simulink subsystem "PackSOC"  (R2021a)
settings: Solver=VariableStepAuto  StartTime=0.0  StopTime=10.0  RelTol=1e-3
undefined symbols (not defined in the file): CDCEstimation, EKFEstimation
settings Model: Creator=mirko  LastModifiedBy=mirko

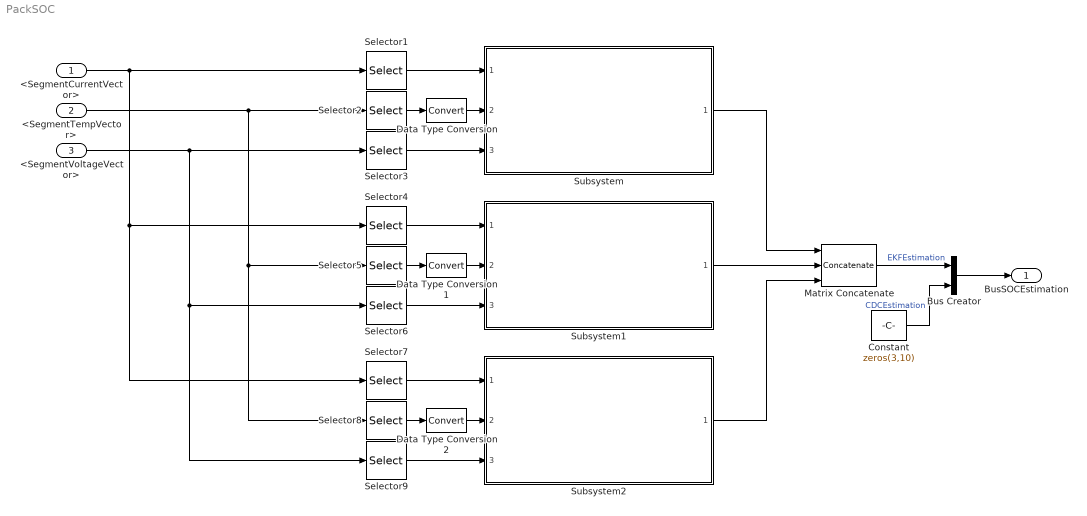
== system PackSOC ==
  <SegmentCurrentVector> : Inport
  <SegmentTempVector> : Inport  Port=2
  <SegmentVoltageVector> : Inport  Port=3
  Bus Creator : BusCreator  Inputs=EKFEstimation,CDCEstimation  OutDataTypeStr=Bus: BusSOCEstimation
  Constant : Constant  Value=zeros(3,10)
  Data Type Conversion : DataTypeConversion
  Data Type Conversion1 : DataTypeConversion
  Data Type Conversion2 : DataTypeConversion
  Matrix Concatenate : Concatenate  NumInputs=3  Mode=Multidimensional array
  Selector1 : Selector  NumberOfDimensions=2  InputPortWidth=3  IndexOptions=Index vector (dialog),Index vector (dialog)  Indices=1,[1 2 3 4 5 6 7 8 9 10]  OutputSizes=1,1
  Selector2 : Selector  NumberOfDimensions=2  InputPortWidth=3  IndexOptions=Index vector (dialog),Index vector (dialog)  Indices=1,[1 2 3 4 5 6 7 8 9 10]  OutputSizes=1,1
  Selector3 : Selector  NumberOfDimensions=2  InputPortWidth=3  IndexOptions=Index vector (dialog),Index vector (dialog)  Indices=1,[1 2 3 4 5 6 7 8 9 10]  OutputSizes=1,1
  Selector4 : Selector  NumberOfDimensions=2  InputPortWidth=3  IndexOptions=Index vector (dialog),Index vector (dialog)  Indices=2,[1 2 3 4 5 6 7 8 9 10]  OutputSizes=1,1
  Selector5 : Selector  NumberOfDimensions=2  InputPortWidth=3  IndexOptions=Index vector (dialog),Index vector (dialog)  Indices=2,[1 2 3 4 5 6 7 8 9 10]  OutputSizes=1,1
  Selector6 : Selector  NumberOfDimensions=2  InputPortWidth=3  IndexOptions=Index vector (dialog),Index vector (dialog)  Indices=2,[1 2 3 4 5 6 7 8 9 10]  OutputSizes=1,1
  Selector7 : Selector  NumberOfDimensions=2  InputPortWidth=3  IndexOptions=Index vector (dialog),Index vector (dialog)  Indices=3,[1 2 3 4 5 6 7 8 9 10]  OutputSizes=1,1
  Selector8 : Selector  NumberOfDimensions=2  InputPortWidth=3  IndexOptions=Index vector (dialog),Index vector (dialog)  Indices=3,[1 2 3 4 5 6 7 8 9 10]  OutputSizes=1,1
  Selector9 : Selector  NumberOfDimensions=2  InputPortWidth=3  IndexOptions=Index vector (dialog),Index vector (dialog)  Indices=3,[1 2 3 4 5 6 7 8 9 10]  OutputSizes=1,1
  Subsystem : Subsystem  ReferencedSubsystem=SegmentSOC
  Subsystem1 : Subsystem  ReferencedSubsystem=SegmentSOC
  Subsystem2 : Subsystem  ReferencedSubsystem=SegmentSOC
  BusSOCEstimation : Outport
  wires:
  <SegmentCurrentVector>/1 -> Selector1/1, Selector7/1, Selector4/1
  <SegmentTempVector>/1 -> Selector2/1, Selector5/1, Selector8/1
  <SegmentVoltageVector>/1 -> Selector3/1, Selector6/1, Selector9/1
  Selector1/1 -> Subsystem/1
  Selector3/1 -> Subsystem/3
  Selector7/1 -> Subsystem2/1
  Selector9/1 -> Subsystem2/3
  Selector4/1 -> Subsystem1/1
  Selector6/1 -> Subsystem1/3
  Subsystem/1 -> Matrix Concatenate/1
  Subsystem1/1 -> Matrix Concatenate/2
  Subsystem2/1 -> Matrix Concatenate/3
  Matrix Concatenate/1 -> Bus Creator/1  "EKFEstimation"
  Bus Creator/1 -> BusSOCEstimation/1
  Constant/1 -> Bus Creator/2  "CDCEstimation"
  Selector2/1 -> Data Type Conversion/1
  Selector8/1 -> Data Type Conversion2/1
  Selector5/1 -> Data Type Conversion1/1
  Data Type Conversion/1 -> Subsystem/2
  Data Type Conversion2/1 -> Subsystem2/2
  Data Type Conversion1/1 -> Subsystem1/2
